simulink model "compressor_model"  (R2021b)
settings: Solver=ode15s  StartTime=0.0  StopTime=1.5*tsim  MinStep=min_step  RelTol=1e-3  AbsTol=1e-3  EnableMultiTasking=on
InitFcn:
  | warning 'off';
values from neighbouring files (symbols this model uses):
  pc_max = 500e3    (= 500000)    [script_compressor.m]
  R_h2 = 4.12    [script_H2_assumption.m]    (also in script_compressor.m; script_init_pressures.m; script_pipe_dim.m; script_refuel.m)
  Tamb = 273.15+10    (= 283.15)    [script_compressor.m]    (also in script_init_pressures.m; script_pipe_dim.m; script_refuel.m)
  Th2_ref = 273.15-65    (= 208.15)    [script_H2_assumption.m]    (also in script_compressor.m = 283; script_refuel.m = (273.15+15)-20*m)
  tsim = 2000    [script_H2_assumption.m]    (also in script_compressor.m; script_init_pressures.m = 10; script_pipe_dim.m = 30; script_refuel.m)
  vch_o = 0.125    [script_compressor.m]    (also in script_init_pressures.m; script_pipe_dim.m; script_refuel.m)
  ws = 1500    [script_compressor.m]
libraries: fl_lib x50, nesl_utility x6, slpidlib x1, fl_ps_legacy_lib x1
(part 1 of 4)
settings Model: Creator=jsagardu  LastModifiedBy=jsagardu
settings SolverCC: AutoScaleAbsTol=off  InitialStep=min_step  AlgebraicLoopSolver=TrustRegion
settings DataIOCC: ReturnWorkspaceOutputs=off
settings OptimizationCC: LifeSpan=inf
settings DebuggingCC: SFUnexpectedBacktrackingDiag=warning  SFNoUnconditionalDefaultTransitionDiag=warning  SFExecutionAtInitializationDiag=none  SFMachineParentedDataDiag=warning  ArithmeticOperatorsInVariantConditions=warning
settings SFSimCC: SimUseLocalCustomCode=off  CustomCodeUndefinedFunction=UseInterfaceOnly
settings RTWCC: RTWUseLocalCustomCode=off
settings CodeAppCC: StateflowObjectComments=on
settings GRTTargetCC: TargetLangStandard=C89/C90 (ANSI)
settings ConfigComp: CovMetricSettings=dw  CovSaveCumulativeToWorkspaceVar=on  CovSaveSingleToWorkspaceVar=on  CovExternalEMLEnable=off
settings SimscapeCC: SimscapeNormalizeSystem=off  SimscapeLogType=local  SimscapeLogLimitData=off  SimscapeLogDataHistory=10000

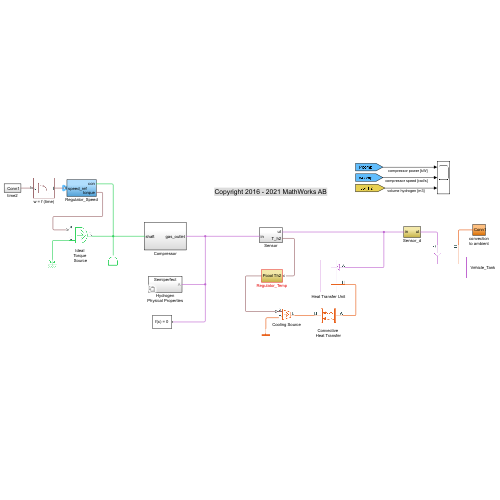
[thumbnail: Simulink's stored preview of the top-level diagram]
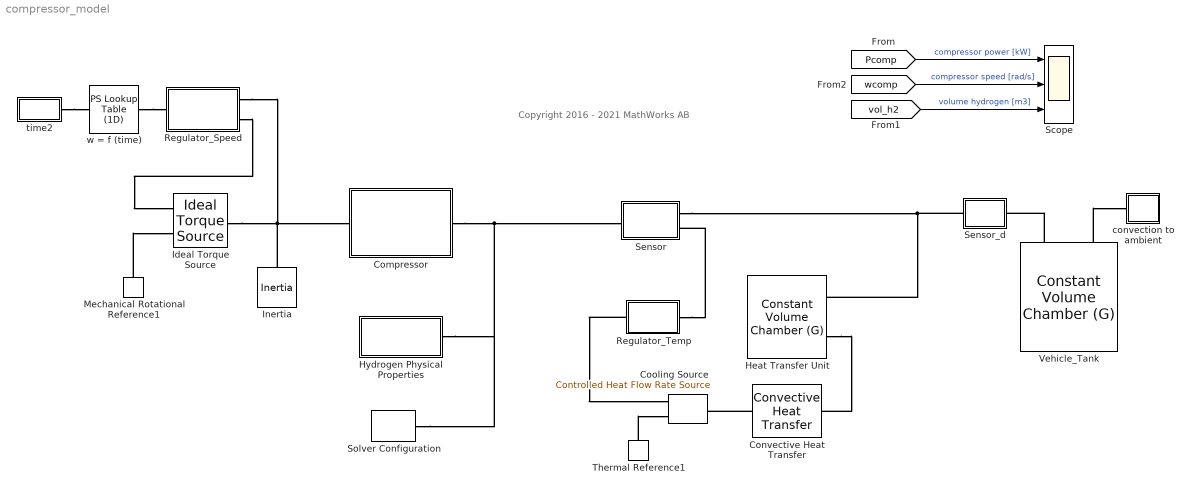
== system compressor_model ==
  note: Copyright 2016 - 2021 MathWorks AB
  Compressor : Subsystem
  Convective Heat Transfer : fl_lib/Thermal/Thermal Elements/Convective Heat Transfer  area=area_ht m^2  heat_tr_coeff=alpha_ht W/(m^2 * K)  T_specify=off  T_priority=None  T=0 K  T_nominal_specify=off  T_nominal_unit=K  T_nominal_value=1  Q_specify=off  Q_priority=None  Q=0 J/s  Q_nominal_specify=off  Q_nominal_unit=W  Q_nominal_value=1
  Cooling Source : fl_lib/Thermal/Thermal Sources/Controlled Heat Flow Rate Source
      settings: LogSimulationData=on
  Heat Transfer Unit : fl_lib/Gas/Elements/Constant Volume Chamber (G)  volume=vol_ht m^3  num_ports=foundation.enum.num_ports.one  area_A=0.01 m^2  area_B=0.01 m^2  area_C=0.01 m^2  area_D=0.01 m^2  p_I_specify=on  p_I_priority=High  p_I=po_init bar  p_I_nominal_specify=off  p_I_nominal_unit=MPa  p_I_nominal_value=1  T_I_specify=on  T_I_priority=High  T_I=To_init K  T_I_nominal_specify=off  T_I_nominal_unit=K  T_I_nominal_value=1  rho_chamber_specify=off  rho_chamber_priority=None  rho_chamber=1.2 kg/m^3  rho_chamber_nominal_specify=off  rho_chamber_nominal_unit=kg/m^3  rho_chamber_nominal_value=1
      settings: SourceProductBaseCode=SS  LogSimulationData=on  InternalSimscapePortConfiguration="{\"Bottom\":[],\"Left\":[{\"id\":\"A\",\"label\":\"A\",\"type\":\"foundation.gas.gas\"},{\"id\":\"H\",\"label\":\"H\",\"type\":\"foundation.thermal.thermal\"}],\"Right\":[],\"Top\":[]}"
  Hydrogen Physical Properties : Subsystem  Variant=on
  Ideal Torque Source : fl_lib/Mechanical/Mechanical Sources/Ideal Torque Source
  Inertia : fl_lib/Mechanical/Rotational Elements/Inertia  inertia=0.05 kg*m^2  num_ports=foundation.enum.numPorts2.one  w_specify=off  w_priority=High  w=0 rad/s  w_nominal_specify=off  w_nominal_unit=rad/s  w_nominal_value=1  t_specify=off  t_priority=None  t=0 N*m  t_nominal_specify=off  t_nominal_unit=N*m  t_nominal_value=1
      settings: LogSimulationData=on
  Mechanical Rotational Reference1 : fl_lib/Mechanical/Rotational Elements/Mechanical Rotational Reference
  Regulator_Speed : Subsystem
  Regulator_Temp : Subsystem
  Scope : Scope  NumInputPorts=3
  Sensor : Subsystem
  Sensor_d : Subsystem
  Solver Configuration : nesl_utility/Solver Configuration  PhysicalDomain=network_engine_domain  SubClassName=solver  LeftPortType=input  RightPortType=generic  Tones=[]  Harmonics=[]  SimulateNoise=off  Profile=off  UseLocalSampling=off  EnableSwitchedLinearOptims=on  FrequencyDomain=off  UseCCode=off  RelTol=0.001  AbsTol=1e-06  MinStep=1e-09  ToWorkspace=off  RevertToSquareIcSolve=off  NumHomotopyIterations=100  PhasorMode=off  PhasorModeNumHarmonics=1  DoDC=off  ResidualTolerance=1e-09  UseLocalSolver=on  LocalSolverChoice=NE_BACKWARD_EULER_ADVANCER  LocalSolverSampleTime=0.1  DoFixedCost=on  MaxNonlinIter=3  MaxModeIter=2  ComputeImpulses=off  ImpulseIterations=2  LinearAlgebra=Sparse  EquationFormulation=NE_TIME_EF  DelaysMemoryBudget=1024  AutomaticFiltering=on  FilteringTimeConstant=0.001  PartitionStorageMethod=AS_NEEDED  PartitionMemoryBudget=1024  PartitionMethod=FAST
      settings: SourceProductBaseCode=PW,SS
  Thermal Reference1 : fl_lib/Thermal/Thermal Elements/Thermal Reference
  Vehicle_Tank : fl_lib/Gas/Elements/Constant Volume Chamber (G)  volume=vch_o m^3  num_ports=foundation.enum.num_ports.one  area_A=0.01 m^2  area_B=0.01 m^2  area_C=0.01 m^2  area_D=0.01 m^2  p_I_specify=off  p_I_priority=High  p_I=1 bar  p_I_nominal_specify=off  p_I_nominal_unit=MPa  p_I_nominal_value=1  T_I_specify=off  T_I_priority=High  T_I=To_init K  T_I_nominal_specify=off  T_I_nominal_unit=K  T_I_nominal_value=1  rho_chamber_specify=off  rho_chamber_priority=None  rho_chamber=1.2 kg/m^3  rho_chamber_nominal_specify=off  rho_chamber_nominal_unit=kg/m^3  rho_chamber_nominal_value=1
      settings: SourceProductBaseCode=SS  LogSimulationData=on  InternalSimscapePortConfiguration="{\"Bottom\":[],\"Left\":[{\"id\":\"A\",\"label\":\"A\",\"type\":\"foundation.gas.gas\"},{\"id\":\"H\",\"label\":\"H\",\"type\":\"foundation.thermal.thermal\"}],\"Right\":[],\"Top\":[]}"
  convection to ambient : Subsystem
  time2 : Subsystem
  w = f (time) : fl_lib/Physical Signals/Lookup Tables/PS Lookup Table (1D)  x=[0 0.55*tsim tsim 1.45*tsim 1.5*tsim] s  f=[0 ws ws 0 0]+(1e-3*ws) rad/s  interp_method=simscape.enum.interpolation.linear  extrap_method=simscape.enum.extrapolation.linear
      settings: SourceProductBaseCode=SS
  wires:
  [Pcomp] -> Scope/1  "compressor power [kW]"
  [vol_h2] -> Scope/3  "volume hydrogen [m3]"
  [wcomp] -> Scope/2  "compressor speed [rad/s]"
  connections:
  Regulator_Speed/LConn1 -- Ideal Torque Source/LConn1 -- Inertia/LConn1 -- Compressor/LConn1
  time2/RConn1 -- w = f (time)/LConn1
  Sensor_d/LConn1 -- Sensor/RConn1 -- Heat Transfer Unit/LConn1
  Convective Heat Transfer/RConn1 -- Cooling Source/LConn1
  Vehicle_Tank/LConn2 -- convection to ambient/LConn1
  Regulator_Temp/LConn1 -- Cooling Source/RConn1
  Heat Transfer Unit/LConn2 -- Convective Heat Transfer/LConn1
  Vehicle_Tank/LConn1 -- Sensor_d/RConn1
  Thermal Reference1/LConn1 -- Cooling Source/RConn2
  Regulator_Temp/RConn1 -- Sensor/RConn2
  Compressor/RConn1 -- Solver Configuration/RConn1 -- Hydrogen Physical Properties/RConn1 -- Sensor/LConn1
  Mechanical Rotational Reference1/LConn1 -- Ideal Torque Source/RConn2
  Regulator_Speed/LConn2 -- Ideal Torque Source/RConn1
  w = f (time)/RConn1 -- Regulator_Speed/RConn1

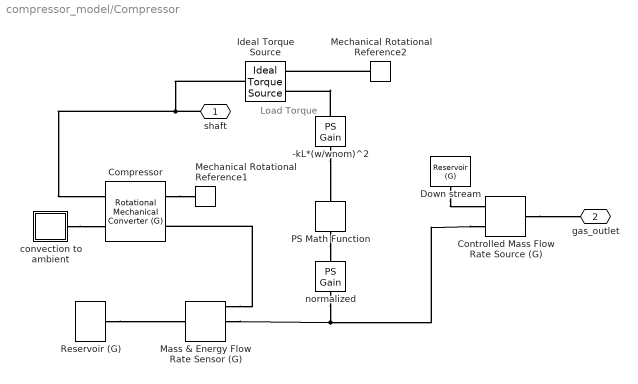
== system compressor_model/Compressor ==
  note: Load Torque
  -kL*(w/wnom)^2 : fl_lib/Physical Signals/Functions/PS Gain  gain=-0.4 N*m
  Compressor : fl_lib/Gas/Elements/Rotational Mechanical Converter (G)  mech_orientation=-1  rotation_spec=foundation.enum.RotationSpec.Calculate  theta_init=0 rad  volume_displacement=disp m^3/rad  dead_volume=1e-5 m^3  area_A=0.01 m^2  environment_spec=1  environment_pressure=0.101325 MPa  p_I_specify=off  p_I_priority=High  p_I=0.101325 MPa  p_I_nominal_specify=off  p_I_nominal_unit=MPa  p_I_nominal_value=1  T_I_specify=off  T_I_priority=High  T_I=293.15 K  T_I_nominal_specify=off  T_I_nominal_unit=K  T_I_nominal_value=1  rho_converter_specify=off  rho_converter_priority=None  rho_converter=1.2 kg/m^3  rho_converter_nominal_specify=off  rho_converter_nominal_unit=kg/m^3  rho_converter_nominal_value=1
      settings: SourceProductBaseCode=SS  LogSimulationData=on  InternalSimscapePortConfiguration="{\"Bottom\":[],\"Left\":[{\"id\":\"A\",\"label\":\"A\",\"type\":\"foundation.gas.gas\"},{\"id\":\"R\",\"label\":\"R\",\"type\":\"foundation.mechanical.rotational.rotational\"}],\"Right\":[{\"id\":\"H\",\"label\":\"H\",\"type\":\"foundation.thermal.thermal\"},{\"id\":\"C\",\"label\":\"C\",\"type\":\"foundation.mechanical.rotational.rotational\"}],\"Top\":[]}"
  Controlled Mass Flow Rate Source (G) : fl_lib/Gas/Sources/Controlled Mass Flow Rate Source (G)  power_spec=foundation.enum.power_spec.isentropic  area_A=0.01 m^2  area_B=0.01 m^2
      settings: SourceProductBaseCode=SS  InternalSimscapePortConfiguration="{\"Bottom\":[],\"Left\":[{\"id\":\"A\",\"label\":\"A\",\"type\":\"foundation.gas.gas\"},{\"id\":\"M\",\"label\":\"M\",\"type\":\"input\"}],\"Right\":[{\"id\":\"B\",\"label\":\"B\",\"type\":\"foundation.gas.gas\"}],\"Top\":[]}"
  Down stream : fl_lib/Gas/Elements/Reservoir (G)  pressure_spec=1  reservoir_pressure=0.101325 MPa  reservoir_temperature=293.15 K  area_A=0.01 m^2
      settings: SourceProductBaseCode=SS  LogSimulationData=on
  Ideal Torque Source : fl_lib/Mechanical/Mechanical Sources/Ideal Torque Source
  Mass & Energy Flow Rate Sensor (G) : fl_lib/Gas/Sensors/Mass & Energy Flow Rate Sensor (G)
      settings: SourceProductBaseCode=SS  InternalSimscapePortConfiguration="{\"Bottom\":[],\"Left\":[{\"id\":\"A\",\"label\":\"A\",\"type\":\"foundation.gas.gas\"}],\"Right\":[{\"id\":\"B\",\"label\":\"B\",\"type\":\"foundation.gas.gas\"},{\"id\":\"M\",\"label\":\"M\",\"type\":\"output\"},{\"id\":\"PHI\",\"label\":\"Phi\",\"type\":\"output\"}],\"Top\":[]}"
  Mechanical Rotational Reference1 : fl_lib/Mechanical/Rotational Elements/Mechanical Rotational Reference
  Mechanical Rotational Reference2 : fl_lib/Mechanical/Rotational Elements/Mechanical Rotational Reference
  PS Math Function : fl_lib/Physical Signals/Functions/PS Math Function  fcn_choice=foundation.enum.math_function.square  v=1
      settings: SourceProductBaseCode=SS
  Reservoir (G) : fl_lib/Gas/Elements/Reservoir (G)  pressure_spec=1  reservoir_pressure=0.101325 MPa  reservoir_temperature=293.15 K  area_A=0.01 m^2
      settings: SourceProductBaseCode=SS  LogSimulationData=on
  convection to ambient : Subsystem
  normalized : fl_lib/Physical Signals/Functions/PS Gain  gain=1/0.0025 1/(kg/s)
  shaft : PMIOPort  Side=Left
  gas_outlet : PMIOPort  Port=2  Side=Right
  connections:
  shaft/RConn1 -- Compressor/RConn2 -- Ideal Torque Source/LConn1
  Controlled Mass Flow Rate Source (G)/RConn1 -- gas_outlet/RConn1
  Reservoir (G)/LConn1 -- Mass & Energy Flow Rate Sensor (G)/LConn1
  convection to ambient/LConn1 -- Compressor/RConn1
  Compressor/LConn2 -- Mechanical Rotational Reference1/LConn1
  Down stream/LConn1 -- Controlled Mass Flow Rate Source (G)/LConn1
  PS Math Function/LConn1 -- normalized/RConn1
  Mass & Energy Flow Rate Sensor (G)/RConn1 -- Compressor/LConn1
  -kL*(w/wnom)^2/LConn1 -- PS Math Function/RConn1
  -kL*(w/wnom)^2/RConn1 -- Ideal Torque Source/RConn1
  Mechanical Rotational Reference2/LConn1 -- Ideal Torque Source/RConn2
  Controlled Mass Flow Rate Source (G)/LConn2 -- normalized/LConn1 -- Mass & Energy Flow Rate Sensor (G)/RConn2

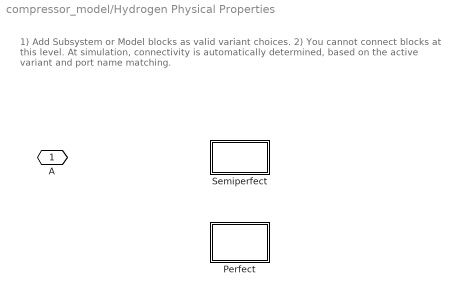
== system compressor_model/Hydrogen Physical Properties ==
  note: 1) Add Subsystem or Model blocks as valid variant choices.
      | 2) You cannot connect blocks at this level. At simulation, connectivity is automatically
      | determined, based on the active variant and port name matching.
  Perfect : Subsystem  VariantControl=var_a>0
  Semiperfect : Subsystem  VariantControl=var_b>0
  A : PMIOPort  Side=Right

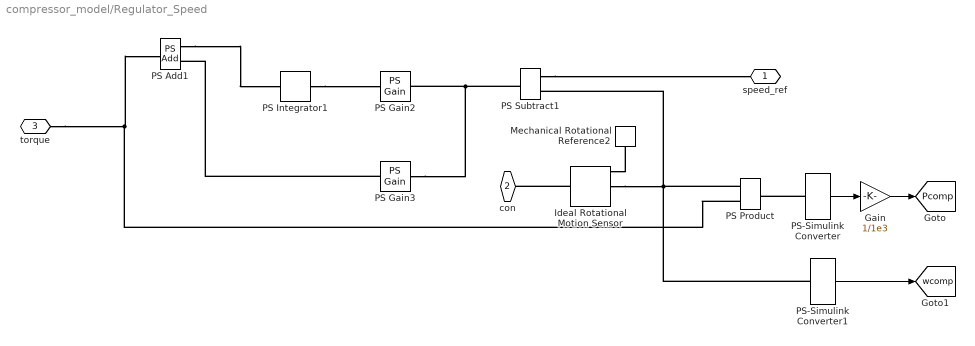
== system compressor_model/Regulator_Speed ==
  Gain : Gain  Gain=1/1e3
  Ideal Rotational Motion Sensor : fl_lib/Mechanical/Mechanical Sensors/Ideal Rotational Motion Sensor  wrap_angle=simscape.enum.onoff.off  offset=0 rad
  Mechanical Rotational Reference2 : fl_lib/Mechanical/Rotational Elements/Mechanical Rotational Reference
  PS Add1 : fl_lib/Physical Signals/Functions/PS Add
  PS Gain2 : fl_lib/Physical Signals/Functions/PS Gain  gain=2.5 N*m/(rad)
  PS Gain3 : fl_lib/Physical Signals/Functions/PS Gain  gain=1 N*m/(rad/s)
  PS Integrator1 : fl_lib/Physical Signals/Linear Operators/PS Integrator  reset_method=foundation.enum.IntegratorResetSpec.None  initial_condition_spec=foundation.enum.IntegratorICSpec.Internal  x0=0 N*m
      settings: SourceProductBaseCode=SS
  PS Product : fl_lib/Physical Signals/Functions/PS Product
  PS Subtract1 : fl_lib/Physical Signals/Functions/PS Subtract
  PS-Simulink Converter : nesl_utility/PS-Simulink Converter  PhysicalDomain=network_engine_domain  SubClassName=ps_output  LeftPortType=input  RightPortType=output  PseudoPeriodic=off  Frequencies=[]  Unit=W  AffineConversion=off
      settings: SourceProductBaseCode=PW,SS
  PS-Simulink Converter1 : nesl_utility/PS-Simulink Converter  PhysicalDomain=network_engine_domain  SubClassName=ps_output  LeftPortType=input  RightPortType=output  PseudoPeriodic=off  Frequencies=[]  Unit=1  AffineConversion=off
      settings: SourceProductBaseCode=PW,SS
  speed_ref : PMIOPort  Side=Right
  con : PMIOPort  Port=2  Side=Left
  torque : PMIOPort  Port=3  Side=Left
  tag scope: Pcomp=global, wcomp=global
  wires:
  PS-Simulink Converter/1 -> Gain/1
  PS-Simulink Converter1/1 -> [wcomp]
  Gain/1 -> [Pcomp]
  connections:
  Ideal Rotational Motion Sensor/RConn2 -- PS Product/LConn1 -- PS-Simulink Converter1/LConn1 -- PS Subtract1/LConn2
  Ideal Rotational Motion Sensor/LConn1 -- con/RConn1
  Ideal Rotational Motion Sensor/RConn1 -- Mechanical Rotational Reference2/LConn1
  PS Subtract1/LConn1 -- speed_ref/RConn1
  PS Integrator1/LConn1 -- PS Gain2/RConn1
  PS Gain3/RConn1 -- PS Add1/LConn2
  PS Add1/LConn1 -- PS Integrator1/RConn1
  PS Subtract1/RConn1 -- PS Gain3/LConn1 -- PS Gain2/LConn1
  torque/RConn1 -- PS Product/LConn2 -- PS Add1/RConn1
  PS-Simulink Converter/LConn1 -- PS Product/RConn1

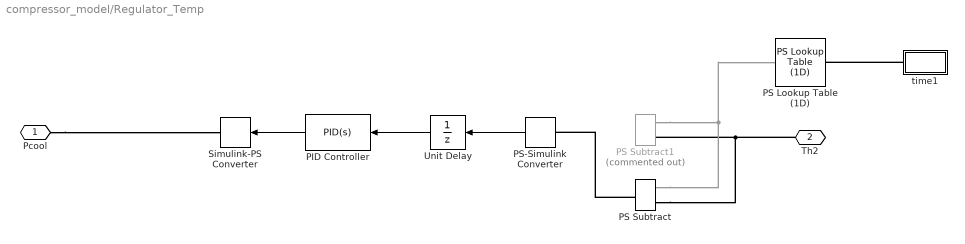
== system compressor_model/Regulator_Temp ==
  PID Controller : slpidlib/PID Controller  Controller=PID  Form=Parallel  TimeDomain=Continuous-time  UseExternalTs=off  SampleTime=-1  IntegratorMethod=Forward Euler  FilterMethod=Forward Euler  ControllerParametersSource=internal  P=36692.3726243318  I=5389.14486996388  D=-310.281463561081  UseFilter=on  N=2.9174592534168  TunerSelectOption=Transfer Function Based (PID Tuner App)  InitialConditionSource=internal  InitialConditionForIntegrator=-pc_max/2  InitialConditionForFilter=0  DifferentiatorICPrevScaledInput=0  ExternalReset=none  TrackingMode=off  Kt=1  LimitOutput=on  SatLimitsSource=internal  UpperSaturationLimit=pc_max  LowerSaturationLimit=-pc_max  LinearizeAsGain=on  AntiWindupMode=back-calculation  Kb=100  POutMin=[]  POutMax=[]  IOutMin=[]  IOutMax=[]  DOutMin=[]  DOutMax=[]  NOutMin=[]  NOutMax=[]  SumOutMin=[]  SumOutMax=[]  SaturationOutMin=[]  SaturationOutMax=[]  PParamMin=[]  PParamMax=[]  IParamMin=[]  IParamMax=[]  DParamMin=[]  DParamMax=[]  NParamMin=[]  NParamMax=[]  KbParamMin=[]  KbParamMax=[]  KtParamMin=[]  KtParamMax=[]  KbOutMin=[]  KbOutMax=[]  KtOutMin=[]  KtOutMax=[]  IntegratorOutMin=[]  IntegratorOutMax=[]  FilterOutMin=[]  FilterOutMax=[]  SumI1OutMin=[]  SumI1OutMax=[]  SumI2OutMin=[]  SumI2OutMax=[]  SumI3OutMin=[]  SumI3OutMax=[]  SumI4OutMin=[]  SumI4OutMax=[]  SumDOutMin=[]  SumDOutMax=[]  DifferentiatorOutMin=[]  DifferentiatorOutMax=[]  FilterDiffOutCoefMin=[]  FilterDiffOutCoefMax=[]  ReciprocalOutMin=[]  ReciprocalOutMax=[]  SumDenOutMin=[]  SumDenOutMax=[]  SumNumOutMin=[]  SumNumOutMax=[]  DivideOutMin=[]  DivideOutMax=[]  UdiffTsProdOutMin=[]  UdiffTsProdOutMax=[]  NTsProdOutMin=[]  NTsProdOutMax=[]  UintegralTsProdOutMin=[]  UintegralTsProdOutMax=[]  UngainTsProdOutMin=[]  UngainTsProdOutMax=[]  IntegratorContinuousStateAttributes=''  IntegratorStateMustResolveToSignalObject=off  IntegratorRTWStateStorageClass=Auto  FilterContinuousStateAttributes=''  FilterStateMustResolveToSignalObject=off  FilterRTWStateStorageClass=Auto  ParallelPVariant=InternalParameters  IdealPVariant=Disabled  IVariant=InternalParameters  DVariant=InternalParameters  IntegratorVariant=Continuous  SatVariant=Enabled  AWVariant=BackCalculation  PCopyVariant=Disabled  TRVariant=Disabled  FdbkBlocksVariant=Forward  IdealPFdbkVariant=Disabled  SatFdbkVariant=Disabled  DerivativeFilterVariant=ContFilter  NVariant=InternalParameters  NCopyVariant=Disabled  FilterICVariant=InternalICsFilter  IntegratorICVariant=InternalICs  ExternalResetVariant=Disabled  TRSumVariant=Passthrough  SumFdbkVariant=Disabled  SumVariant=Sum_PID  TsampFilterVariant=InternalTs  TsampNgainVariant=Passthrough  TsampIntegralVariant=Passthrough  ExternalSaturationOutDataTypeStr=Inherit: Same as second input
  PS Lookup Table (1D) : fl_lib/Physical Signals/Lookup Tables/PS Lookup Table (1D)  x=[0 500 tsim] s  f=273.15+[0 1 1]*(Th2_ref-Tamb) K  interp_method=simscape.enum.interpolation.linear  extrap_method=simscape.enum.extrapolation.linear
      settings: SourceProductBaseCode=SS
  PS Subtract : fl_lib/Physical Signals/Functions/PS Subtract
  PS Subtract1 : fl_ps_legacy_lib/Legacy Physical Signals/Functions/PS Subtract  Commented=on
      settings: SourceProductBaseCode=SS
  PS-Simulink Converter : nesl_utility/PS-Simulink Converter  PhysicalDomain=network_engine_domain  SubClassName=ps_output  LeftPortType=input  RightPortType=output  PseudoPeriodic=off  Frequencies=[]  Unit=K  AffineConversion=off
      settings: SourceProductBaseCode=PW,SS
  Simulink-PS Converter : nesl_utility/Simulink-PS Converter  PhysicalDomain=network_engine_domain  SubClassName=ps_input  LeftPortType=input  RightPortType=output  PseudoPeriodic=off  Frequencies=[]  NoiseDistribution=none  NoiseParameters=[]  Unit=1  AffineConversion=off  FilteringAndDerivatives=zero  SimscapeFilterOrder=1  InputFilterTimeConstant=0.5  UdotUserProvided=1
      settings: SourceProductBaseCode=PW,SS
  Unit Delay : UnitDelay  InitialCondition=125  SampleTime=0.1  HasFrameUpgradeWarning=on
  time1 : Subsystem
  Pcool : PMIOPort  Side=Left
  Th2 : PMIOPort  Port=2  Side=Right
  wires:
  PID Controller/1 -> Simulink-PS Converter/1
  PS-Simulink Converter/1 -> Unit Delay/1
  Unit Delay/1 -> PID Controller/1
  connections:
  Pcool/RConn1 -- Simulink-PS Converter/RConn1
  Th2/RConn1 -- PS Subtract/LConn2 -- PS Subtract1/LConn2
  time1/RConn1 -- PS Lookup Table (1D)/LConn1
  PS Subtract1/LConn1 -- PS Lookup Table (1D)/RConn1 -- PS Subtract/LConn1
  PS Subtract/RConn1 -- PS-Simulink Converter/LConn1

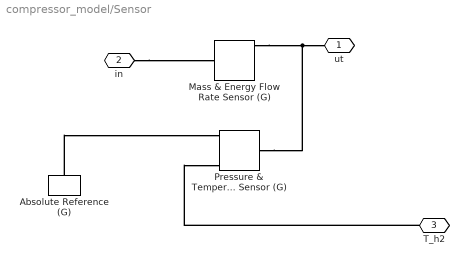
== system compressor_model/Sensor ==
  Absolute Reference (G) : fl_lib/Gas/Elements/Absolute Reference (G)
      settings: SourceProductBaseCode=SS  InternalSimscapePortConfiguration="{\"Bottom\":[],\"Left\":[{\"id\":\"A\",\"label\":\"\",\"type\":\"foundation.gas.gas\"}],\"Right\":[],\"Top\":[]}"
  Mass & Energy Flow Rate Sensor (G) : fl_lib/Gas/Sensors/Mass & Energy Flow Rate Sensor (G)
      settings: SourceProductBaseCode=SS  InternalSimscapePortConfiguration="{\"Bottom\":[],\"Left\":[{\"id\":\"A\",\"label\":\"A\",\"type\":\"foundation.gas.gas\"}],\"Right\":[{\"id\":\"B\",\"label\":\"B\",\"type\":\"foundation.gas.gas\"},{\"id\":\"M\",\"label\":\"M\",\"type\":\"output\"},{\"id\":\"PHI\",\"label\":\"Phi\",\"type\":\"output\"}],\"Top\":[]}"
  Pressure & Temperature Sensor (G) : fl_lib/Gas/Sensors/Pressure & Temperature Sensor (G)
      settings: SourceProductBaseCode=SS  LogSimulationData=on  InternalSimscapePortConfiguration="{\"Bottom\":[],\"Left\":[{\"id\":\"A\",\"label\":\"A\",\"type\":\"foundation.gas.gas\"}],\"Right\":[{\"id\":\"B\",\"label\":\"B\",\"type\":\"foundation.gas.gas\"},{\"id\":\"P\",\"label\":\"P\",\"type\":\"output\"},{\"id\":\"T\",\"label\":\"T\",\"type\":\"output\"}],\"Top\":[]}"
  ut : PMIOPort  Side=Right
  in : PMIOPort  Port=2  Side=Left
  T_h2 : PMIOPort  Port=3  Side=Right
  connections:
  Absolute Reference (G)/LConn1 -- Pressure & Temperature Sensor (G)/RConn1
  in/RConn1 -- Mass & Energy Flow Rate Sensor (G)/LConn1
  Mass & Energy Flow Rate Sensor (G)/RConn1 -- Pressure & Temperature Sensor (G)/LConn1 -- ut/RConn1
  T_h2/RConn1 -- Pressure & Temperature Sensor (G)/RConn3

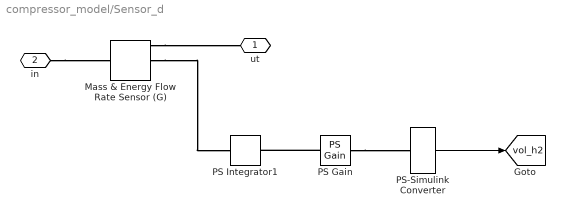
== system compressor_model/Sensor_d ==
  Mass & Energy Flow Rate Sensor (G) : fl_lib/Gas/Sensors/Mass & Energy Flow Rate Sensor (G)
      settings: SourceProductBaseCode=SS  InternalSimscapePortConfiguration="{\"Bottom\":[],\"Left\":[{\"id\":\"A\",\"label\":\"A\",\"type\":\"foundation.gas.gas\"}],\"Right\":[{\"id\":\"B\",\"label\":\"B\",\"type\":\"foundation.gas.gas\"},{\"id\":\"M\",\"label\":\"M\",\"type\":\"output\"},{\"id\":\"PHI\",\"label\":\"Phi\",\"type\":\"output\"}],\"Top\":[]}"
  PS Gain : fl_lib/Physical Signals/Functions/PS Gain  gain=1/vch_o m^3/kg
  PS Integrator1 : fl_lib/Physical Signals/Linear Operators/PS Integrator  reset_method=foundation.enum.IntegratorResetSpec.None  initial_condition_spec=foundation.enum.IntegratorICSpec.Internal  x0=0 kg
      settings: SourceProductBaseCode=SS
  PS-Simulink Converter : nesl_utility/PS-Simulink Converter  PhysicalDomain=network_engine_domain  SubClassName=ps_output  LeftPortType=input  RightPortType=output  PseudoPeriodic=off  Frequencies=[]  Unit=m^3  AffineConversion=off
      settings: SourceProductBaseCode=PW,SS
  ut : PMIOPort  Side=Right
  in : PMIOPort  Port=2  Side=Left
  tag scope: vol_h2=global
  wires:
  PS-Simulink Converter/1 -> [vol_h2]
  connections:
  Mass & Energy Flow Rate Sensor (G)/RConn2 -- PS Integrator1/LConn1
  Mass & Energy Flow Rate Sensor (G)/RConn1 -- ut/RConn1
  in/RConn1 -- Mass & Energy Flow Rate Sensor (G)/LConn1
  PS Gain/RConn1 -- PS-Simulink Converter/LConn1
  PS Gain/LConn1 -- PS Integrator1/RConn1

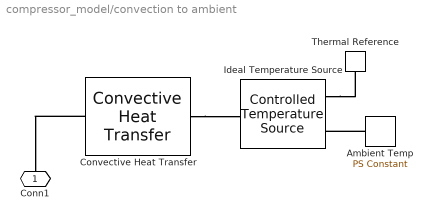
== system compressor_model/convection to ambient ==
  Ambient Temp : fl_lib/Physical Signals/Sources/PS Constant  constant=Tamb
  Convective Heat Transfer : fl_lib/Thermal/Thermal Elements/Convective Heat Transfer  area=1e-4 m^2  heat_tr_coeff=alpha W/(m^2 * K)  T_specify=off  T_priority=None  T=0 K  T_nominal_specify=off  T_nominal_unit=K  T_nominal_value=1  Q_specify=off  Q_priority=None  Q=0 J/s  Q_nominal_specify=off  Q_nominal_unit=W  Q_nominal_value=1
  Ideal Temperature Source : fl_lib/Thermal/Thermal Sources/Controlled Temperature Source
  Thermal Reference : fl_lib/Thermal/Thermal Elements/Thermal Reference
  Conn1 : PMIOPort  Side=Left
  connections:
  Ambient Temp/RConn1 -- Ideal Temperature Source/RConn1
  Ideal Temperature Source/RConn2 -- Thermal Reference/LConn1
  Convective Heat Transfer/LConn1 -- Conn1/RConn1
  Convective Heat Transfer/RConn1 -- Ideal Temperature Source/LConn1

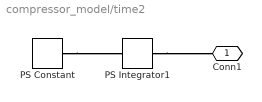
== system compressor_model/time2 ==
  PS Constant : fl_lib/Physical Signals/Sources/PS Constant  constant=1
  PS Integrator1 : fl_lib/Physical Signals/Linear Operators/PS Integrator  reset_method=foundation.enum.IntegratorResetSpec.None  initial_condition_spec=foundation.enum.IntegratorICSpec.Internal  x0=0 s
      settings: SourceProductBaseCode=SS
  Conn1 : PMIOPort  Side=Right
  connections:
  PS Integrator1/RConn1 -- Conn1/RConn1
  PS Constant/RConn1 -- PS Integrator1/LConn1

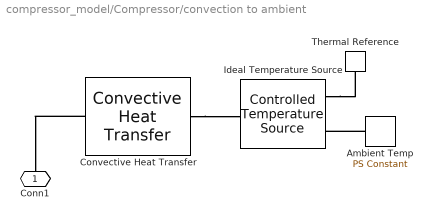
== system compressor_model/Compressor/convection to ambient ==
  Ambient Temp : fl_lib/Physical Signals/Sources/PS Constant  constant=Tamb
  Convective Heat Transfer : fl_lib/Thermal/Thermal Elements/Convective Heat Transfer  area=0.25 m^2  heat_tr_coeff=alpha W/(m^2 * K)  T_specify=off  T_priority=None  T=0 K  T_nominal_specify=off  T_nominal_unit=K  T_nominal_value=1  Q_specify=off  Q_priority=None  Q=0 J/s  Q_nominal_specify=off  Q_nominal_unit=W  Q_nominal_value=1
  Ideal Temperature Source : fl_lib/Thermal/Thermal Sources/Controlled Temperature Source
  Thermal Reference : fl_lib/Thermal/Thermal Elements/Thermal Reference
  Conn1 : PMIOPort  Side=Left
  connections:
  Ambient Temp/RConn1 -- Ideal Temperature Source/RConn1
  Ideal Temperature Source/RConn2 -- Thermal Reference/LConn1
  Convective Heat Transfer/LConn1 -- Conn1/RConn1
  Convective Heat Transfer/RConn1 -- Ideal Temperature Source/LConn1
